simulink model "Adelanto_digital_tarea"  (R2021a)
settings: Solver=ode45  StartTime=0.0  StopTime=10  MaxStep=1e-5  RelTol=1e-3  EnableMultiTasking=on
values from neighbouring files (symbols this model uses):
  c = 0.52-d    [Pruebas.m]
  p1 = 0.52+j*0.43    [Pruebas.m]    (also in Tp2.m = 0.7851+j*0.2361)
  T = 0.2    [Pruebas.m]
undefined symbols (not defined in the file or in its folder): cc, K, Kc, p2, pc
settings Model: Creator=Usuario  LastModifiedBy=bruno
settings SolverCC: AlgebraicLoopSolver=TrustRegion
settings DataIOCC: SaveFormat=Array  SignalLoggingSaveFormat=ModelDataLogs  ReturnWorkspaceOutputs=off
settings OptimizationCC: InitFltsAndDblsToZero=on  LifeSpan=inf
settings DebuggingCC: SaveWithParameterizedLinksMsg=none  UnderspecifiedInitializationDetection=Classic  MergeDetectMultiDrivingBlocksExec=none  SignalResolutionControl=TryResolveAllWithWarning  SolverPrmCheckMsg=warning  MultiTaskDSMMsg=warning  MultiTaskCondExecSysMsg=none  FcnCallInpInsideContextMsg=warning  SFUnexpectedBacktrackingDiag=warning  SFNoUnconditionalDefaultTransitionDiag=warning  SFExecutionAtInitializationDiag=none  SFMachineParentedDataDiag=warning  ArithmeticOperatorsInVariantConditions=warning
settings HardwareCC: ProdBitPerPointer=32  ProdBitPerSizeT=32  ProdBitPerPtrDiffT=32  ProdLargestAtomicFloat=None  ProdIntDivRoundTo=Undefined  ProdEndianess=Unspecified  ProdWordSize=32  ProdHWDeviceType=32-bit Generic
settings ModelReferenceCC: PropagateSignalLabelsOutOfModel=off
settings SFSimCC: SimUseLocalCustomCode=off  CustomCodeUndefinedFunction=UseInterfaceOnly
settings RTWCC: RTWUseLocalCustomCode=off
settings CodeAppCC: StateflowObjectComments=on
settings GRTTargetCC: TargetFcnLib=ansi_tfl_tmw.mat  TargetLangStandard=C89/C90 (ANSI)  CombineOutputUpdateFcns=off  GRTInterface=on
settings ConfigComp: CovMetricSettings=dw  CovSaveCumulativeToWorkspaceVar=on  CovSaveSingleToWorkspaceVar=on  CovExternalEMLEnable=off  CovSFcnEnable=off

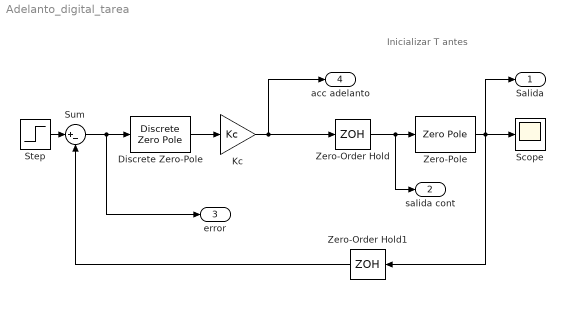
== system Adelanto_digital_tarea ==
  note: Inicializar T antes
  Discrete Zero-Pole : DiscreteZeroPole  Zeros=[cc]  Poles=[pc]  Gain=1  SampleTime=-1
  Kc : Gain  Gain=Kc
  Scope : Scope
  Step : Step  Time=0  SampleTime=T
  Sum : Sum  Inputs=|+-
  Zero-Order Hold : ZeroOrderHold  SampleTime=T
  Zero-Order Hold1 : ZeroOrderHold  SampleTime=T
  Zero-Pole : ZeroPole  Zeros=[c]  Poles=[p1 p2]  Gain=[K]
  Salida : Outport
  salida cont : Outport  Port=2
  error : Outport  Port=3
  acc adelanto : Outport  Port=4
  wires:
  Zero-Order Hold/1 -> Zero-Pole/1, salida cont/1
  Step/1 -> Sum/1
  Zero-Pole/1 -> Zero-Order Hold1/1, Scope/1, Salida/1
  Zero-Order Hold1/1 -> Sum/2
  Sum/1 -> Discrete Zero-Pole/1, error/1
  Kc/1 -> Zero-Order Hold/1, acc adelanto/1
  Discrete Zero-Pole/1 -> Kc/1
